simulink model "ArduCopter_3DR"  (R2015a)
settings: Solver=ode45  StartTime=0.0  StopTime=10.0  RelTol=1e-3
settings Model: CovModelRefEnable=off  Creator=pa872d  LastModifiedBy=anne

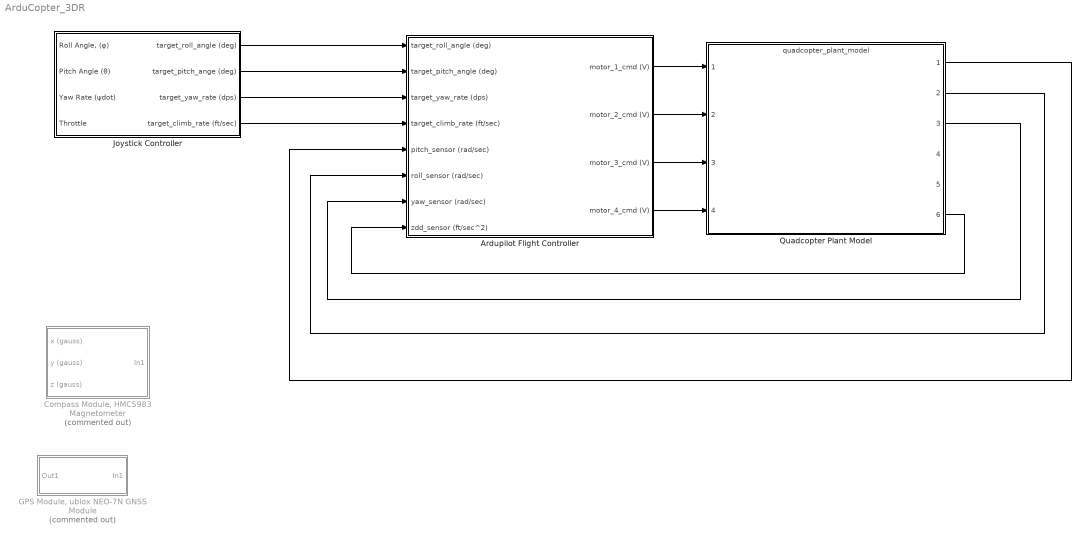
== system ArduCopter_3DR ==
  Ardupilot Flight Controller : Subsystem
  "Compass Module, HMC5983 Magnetometer" : Subsystem  Commented=on
  "GPS Module, ublox NEO-7N GNSS Module" : Subsystem  Commented=on
  Joystick Controller : Subsystem
  Quadcopter Plant Model : ModelReference  ModelNameDialog=quadcopter_plant_model.slx  SimulationMode=Normal  ModelReferenceVersion=1.2  CopyOfModelName=attitude_controller.slx  CopyOfModelName=motor_mixer.slx
  wires:
  Joystick Controller/1(target_roll_angle (deg)) -> Ardupilot Flight Controller/1(target_roll_angle (deg))
  Joystick Controller/2(target_pitch_ange (deg)) -> Ardupilot Flight Controller/2(target_pitch_angle (deg))
  Joystick Controller/3(target_yaw_rate (dps)) -> Ardupilot Flight Controller/3(target_yaw_rate (dps))
  Joystick Controller/4(target_climb_rate (ft/sec)) -> Ardupilot Flight Controller/4(target_climb_rate (ft/sec))
  Quadcopter Plant Model/1 -> Ardupilot Flight Controller/5(pitch_sensor (rad/sec))
  Quadcopter Plant Model/3 -> Ardupilot Flight Controller/7(yaw_sensor (rad/sec))
  Ardupilot Flight Controller/1(motor_1_cmd (V)) -> Quadcopter Plant Model/1
  Ardupilot Flight Controller/2(motor_2_cmd (V)) -> Quadcopter Plant Model/2
  Ardupilot Flight Controller/3(motor_3_cmd (V)) -> Quadcopter Plant Model/3
  Ardupilot Flight Controller/4(motor_4_cmd (V)) -> Quadcopter Plant Model/4
  Quadcopter Plant Model/2 -> Ardupilot Flight Controller/6(roll_sensor (rad/sec))
  Quadcopter Plant Model/6 -> Ardupilot Flight Controller/8(zdd_sensor (ft/sec^2))

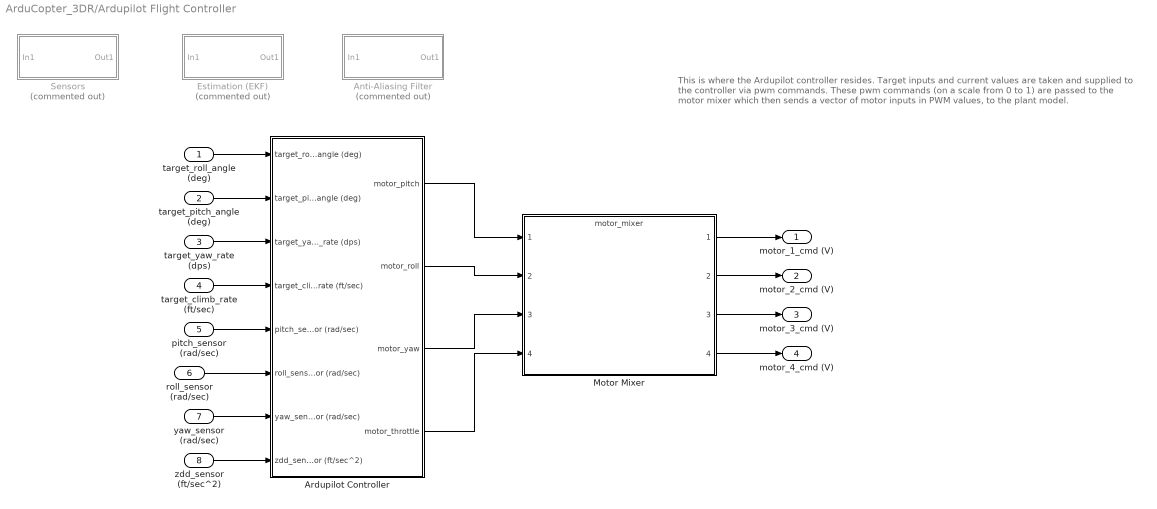
== system ArduCopter_3DR/Ardupilot Flight Controller ==
  note: This is where the Ardupilot controller resides. Target inputs and current values are taken and
      | supplied to the controller via pwm commands. These pwm commands (on a scale from 0 to 1) are passed to the motor mixer which then
      | sends a vector of motor inputs in PWM values, to the plant model.
  target_roll_angle (deg) : Inport
  target_pitch_angle (deg) : Inport  Port=2
  target_yaw_rate (dps) : Inport  Port=3
  target_climb_rate (ft/sec) : Inport  Port=4
  pitch_sensor (rad/sec) : Inport  Port=5
  roll_sensor (rad/sec) : Inport  Port=6
  yaw_sensor (rad/sec) : Inport  Port=7
  zdd_sensor (ft/sec^2) : Inport  Port=8
  Anti-Aliasing Filter : Subsystem  Commented=on
  Ardupilot Controller : Subsystem
  Estimation (EKF) : Subsystem  Commented=on
  Motor Mixer : ModelReference  ModelNameDialog=motor_mixer.slx  SimulationMode=Normal  ModelReferenceVersion=1.6  CopyOfModelName=attitude_controller.slx  CopyOfModelName=motor_mixer.slx
  Sensors : Subsystem  Commented=on
  motor_1_cmd (V) : Outport
  motor_2_cmd (V) : Outport  Port=2
  motor_3_cmd (V) : Outport  Port=3
  motor_4_cmd (V) : Outport  Port=4
  wires:
  Motor Mixer/2 -> motor_2_cmd (V)/1
  Motor Mixer/4 -> motor_4_cmd (V)/1
  Motor Mixer/3 -> motor_3_cmd (V)/1
  target_roll_angle (deg)/1 -> Ardupilot Controller/1(target_roll_angle (deg))
  target_pitch_angle (deg)/1 -> Ardupilot Controller/2(target_pitch_angle (deg))
  target_yaw_rate (dps)/1 -> Ardupilot Controller/3(target_yaw_rate (dps))
  target_climb_rate (ft/sec)/1 -> Ardupilot Controller/4(target_climb_rate (ft/sec))
  Motor Mixer/1 -> motor_1_cmd (V)/1
  yaw_sensor (rad/sec)/1 -> Ardupilot Controller/7(yaw_sensor (rad/sec))
  zdd_sensor (ft/sec^2)/1 -> Ardupilot Controller/8(zdd_sensor (ft/sec^2))
  Ardupilot Controller/1(motor_pitch) -> Motor Mixer/1
  Ardupilot Controller/2(motor_roll) -> Motor Mixer/2
  Ardupilot Controller/3(motor_yaw) -> Motor Mixer/3
  Ardupilot Controller/4(motor_throttle) -> Motor Mixer/4
  roll_sensor (rad/sec)/1 -> Ardupilot Controller/6(roll_sensor (rad/sec))
  pitch_sensor (rad/sec)/1 -> Ardupilot Controller/5(pitch_sensor (rad/sec))

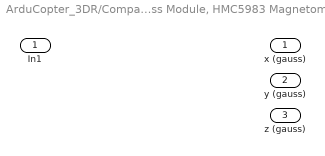
== system ArduCopter_3DR/Compass Module, HMC5983 Magnetometer ==
  In1 : Inport
  x (gauss) : Outport
  y (gauss) : Outport  Port=2
  z (gauss) : Outport  Port=3

== system ArduCopter_3DR/GPS Module, ublox NEO-7N GNSS Module ==
  In1 : Inport
  Out1 : Outport
  wires:
  In1/1 -> Out1/1

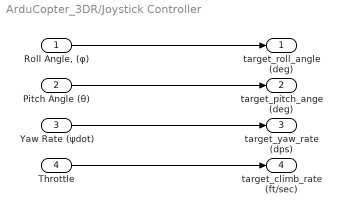
== system ArduCopter_3DR/Joystick Controller ==
  "Roll Angle, (φ)" : Inport
  Pitch Angle (θ) : Inport  Port=2
  Yaw Rate (ψdot) : Inport  Port=3
  Throttle : Inport  Port=4
  target_roll_angle (deg) : Outport
  target_pitch_ange (deg) : Outport  Port=2
  target_yaw_rate (dps) : Outport  Port=3
  target_climb_rate (ft/sec) : Outport  Port=4
  wires:
  Yaw Rate (ψdot)/1 -> target_yaw_rate (dps)/1
  Throttle/1 -> target_climb_rate (ft/sec)/1
  Pitch Angle (θ)/1 -> target_pitch_ange (deg)/1
  "Roll Angle, (φ)"/1 -> target_roll_angle (deg)/1

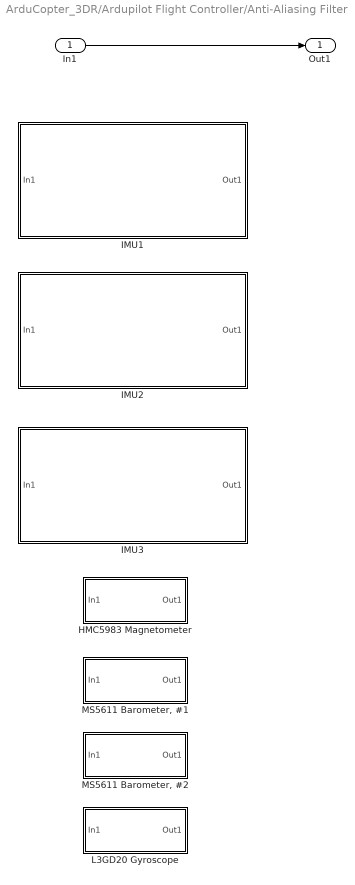
== system ArduCopter_3DR/Ardupilot Flight Controller/Anti-Aliasing Filter ==
  In1 : Inport
  HMC5983 Magnetometer : Subsystem
  IMU1 : Subsystem
  IMU2 : Subsystem
  IMU3 : Subsystem
  L3GD20 Gyroscope : Subsystem
  "MS5611 Barometer, #1" : Subsystem
  "MS5611 Barometer, #2" : Subsystem
  Out1 : Outport
  wires:
  In1/1 -> Out1/1

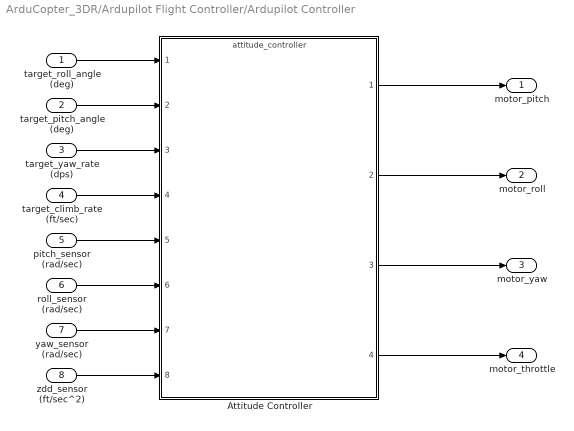
== system ArduCopter_3DR/Ardupilot Flight Controller/Ardupilot Controller ==
  target_roll_angle (deg) : Inport
  target_pitch_angle (deg) : Inport  Port=2
  target_yaw_rate (dps) : Inport  Port=3
  target_climb_rate (ft/sec) : Inport  Port=4
  pitch_sensor (rad/sec) : Inport  Port=5
  roll_sensor (rad/sec) : Inport  Port=6
  yaw_sensor (rad/sec) : Inport  Port=7
  zdd_sensor (ft/sec^2) : Inport  Port=8
  Attitude Controller : ModelReference  ModelNameDialog=attitude_controller.slx  SimulationMode=Normal  ModelReferenceVersion=1.62  CopyOfModelName=attitude_controller.slx  CopyOfModelName=motor_mixer.slx
  motor_pitch : Outport
  motor_roll : Outport  Port=2
  motor_yaw : Outport  Port=3
  motor_throttle : Outport  Port=4
  wires:
  Attitude Controller/4 -> motor_throttle/1
  Attitude Controller/3 -> motor_yaw/1
  target_roll_angle (deg)/1 -> Attitude Controller/1
  target_pitch_angle (deg)/1 -> Attitude Controller/2
  target_yaw_rate (dps)/1 -> Attitude Controller/3
  target_climb_rate (ft/sec)/1 -> Attitude Controller/4
  yaw_sensor (rad/sec)/1 -> Attitude Controller/7
  zdd_sensor (ft/sec^2)/1 -> Attitude Controller/8
  roll_sensor (rad/sec)/1 -> Attitude Controller/6
  pitch_sensor (rad/sec)/1 -> Attitude Controller/5
  Attitude Controller/2 -> motor_roll/1
  Attitude Controller/1 -> motor_pitch/1

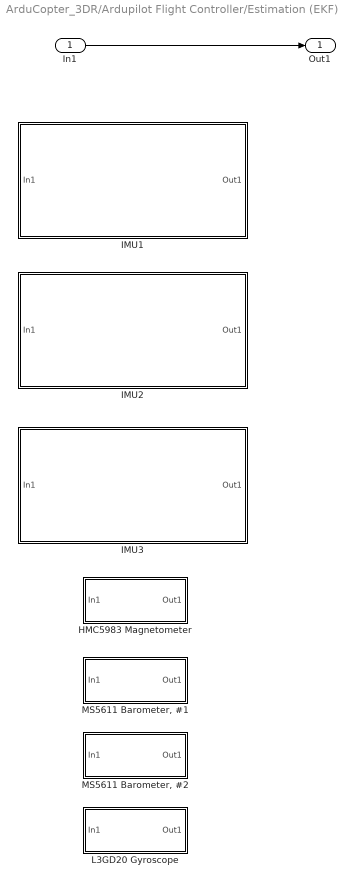
== system ArduCopter_3DR/Ardupilot Flight Controller/Estimation (EKF) ==
  In1 : Inport
  HMC5983 Magnetometer : Subsystem
  IMU1 : Subsystem
  IMU2 : Subsystem
  IMU3 : Subsystem
  L3GD20 Gyroscope : Subsystem
  "MS5611 Barometer, #1" : Subsystem
  "MS5611 Barometer, #2" : Subsystem
  Out1 : Outport
  wires:
  In1/1 -> Out1/1

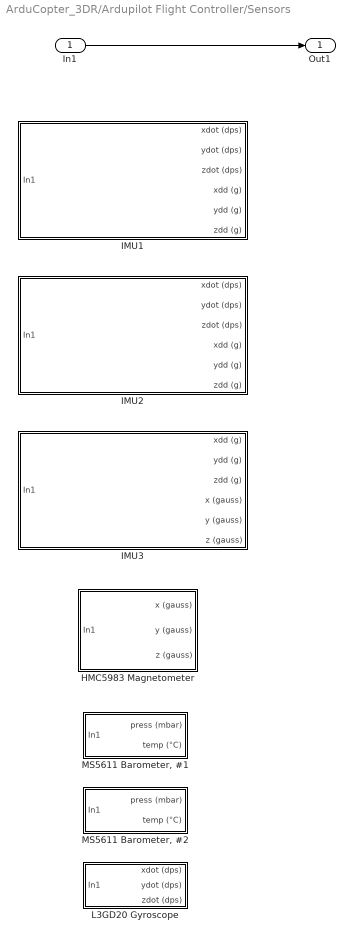
== system ArduCopter_3DR/Ardupilot Flight Controller/Sensors ==
  In1 : Inport
  HMC5983 Magnetometer : Subsystem
  IMU1 : Subsystem
  IMU2 : Subsystem
  IMU3 : Subsystem
  L3GD20 Gyroscope : Subsystem
  "MS5611 Barometer, #1" : Subsystem
  "MS5611 Barometer, #2" : Subsystem
  Out1 : Outport
  wires:
  In1/1 -> Out1/1

== system ArduCopter_3DR/Ardupilot Flight Controller/Anti-Aliasing Filter/HMC5983 Magnetometer ==
  In1 : Inport
  Out1 : Outport
  wires:
  In1/1 -> Out1/1

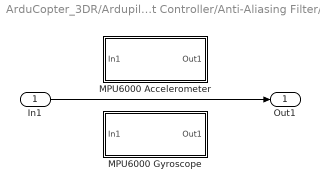
== system ArduCopter_3DR/Ardupilot Flight Controller/Anti-Aliasing Filter/IMU1 ==
  In1 : Inport
  MPU6000 Accelerometer : Subsystem
  MPU6000 Gyroscope : Subsystem
  Out1 : Outport
  wires:
  In1/1 -> Out1/1

== system ArduCopter_3DR/Ardupilot Flight Controller/Anti-Aliasing Filter/IMU2 ==
  In1 : Inport
  MPU6000 Accelerometer : Subsystem
  MPU6000 Gyroscope : Subsystem
  Out1 : Outport
  wires:
  In1/1 -> Out1/1

== system ArduCopter_3DR/Ardupilot Flight Controller/Anti-Aliasing Filter/IMU3 ==
  In1 : Inport
  LSM303D Accelerometer : Subsystem
  LSM303D Magnetometer : Subsystem
  Out1 : Outport
  wires:
  In1/1 -> Out1/1

== system ArduCopter_3DR/Ardupilot Flight Controller/Anti-Aliasing Filter/L3GD20 Gyroscope ==
  In1 : Inport
  Out1 : Outport
  wires:
  In1/1 -> Out1/1

== system ArduCopter_3DR/Ardupilot Flight Controller/Anti-Aliasing Filter/MS5611 Barometer, #1 ==
  In1 : Inport
  Out1 : Outport
  wires:
  In1/1 -> Out1/1

== system ArduCopter_3DR/Ardupilot Flight Controller/Anti-Aliasing Filter/MS5611 Barometer, #2 ==
  In1 : Inport
  Out1 : Outport
  wires:
  In1/1 -> Out1/1

== system ArduCopter_3DR/Ardupilot Flight Controller/Estimation (EKF)/HMC5983 Magnetometer ==
  In1 : Inport
  Out1 : Outport
  wires:
  In1/1 -> Out1/1

== system ArduCopter_3DR/Ardupilot Flight Controller/Estimation (EKF)/IMU1 ==
  In1 : Inport
  MPU6000 Accelerometer : Subsystem
  MPU6000 Gyroscope : Subsystem
  Out1 : Outport
  wires:
  In1/1 -> Out1/1

== system ArduCopter_3DR/Ardupilot Flight Controller/Estimation (EKF)/IMU2 ==
  In1 : Inport
  MPU6000 Accelerometer : Subsystem
  MPU6000 Gyroscope : Subsystem
  Out1 : Outport
  wires:
  In1/1 -> Out1/1

== system ArduCopter_3DR/Ardupilot Flight Controller/Estimation (EKF)/IMU3 ==
  In1 : Inport
  LSM303D Accelerometer : Subsystem
  LSM303D Magnetometer : Subsystem
  Out1 : Outport
  wires:
  In1/1 -> Out1/1

== system ArduCopter_3DR/Ardupilot Flight Controller/Estimation (EKF)/L3GD20 Gyroscope ==
  In1 : Inport
  Out1 : Outport
  wires:
  In1/1 -> Out1/1

== system ArduCopter_3DR/Ardupilot Flight Controller/Estimation (EKF)/MS5611 Barometer, #1 ==
  In1 : Inport
  Out1 : Outport
  wires:
  In1/1 -> Out1/1

== system ArduCopter_3DR/Ardupilot Flight Controller/Estimation (EKF)/MS5611 Barometer, #2 ==
  In1 : Inport
  Out1 : Outport
  wires:
  In1/1 -> Out1/1

== system ArduCopter_3DR/Ardupilot Flight Controller/Sensors/HMC5983 Magnetometer ==
  In1 : Inport
  x (gauss) : Outport
  y (gauss) : Outport  Port=2
  z (gauss) : Outport  Port=3

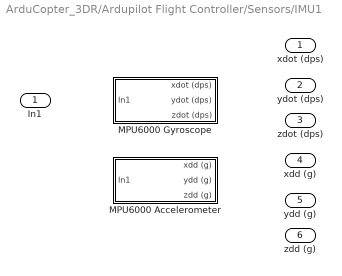
== system ArduCopter_3DR/Ardupilot Flight Controller/Sensors/IMU1 ==
  In1 : Inport
  MPU6000 Accelerometer : Subsystem
  MPU6000 Gyroscope : Subsystem
  xdot (dps) : Outport
  ydot (dps) : Outport  Port=2
  zdot (dps) : Outport  Port=3
  xdd (g) : Outport  Port=4
  ydd (g) : Outport  Port=5
  zdd (g) : Outport  Port=6

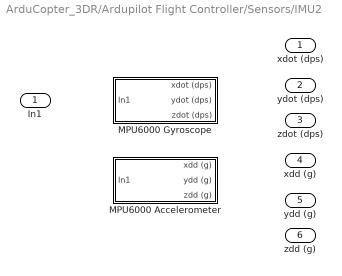
== system ArduCopter_3DR/Ardupilot Flight Controller/Sensors/IMU2 ==
  In1 : Inport
  MPU6000 Accelerometer : Subsystem
  MPU6000 Gyroscope : Subsystem
  xdot (dps) : Outport
  ydot (dps) : Outport  Port=2
  zdot (dps) : Outport  Port=3
  xdd (g) : Outport  Port=4
  ydd (g) : Outport  Port=5
  zdd (g) : Outport  Port=6

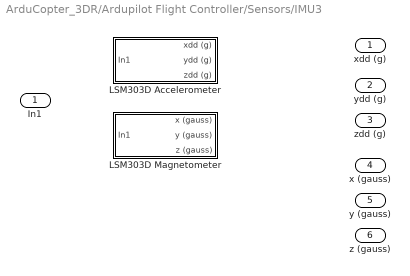
== system ArduCopter_3DR/Ardupilot Flight Controller/Sensors/IMU3 ==
  In1 : Inport
  LSM303D Accelerometer : Subsystem
  LSM303D Magnetometer : Subsystem
  xdd (g) : Outport
  ydd (g) : Outport  Port=2
  zdd (g) : Outport  Port=3
  x (gauss) : Outport  Port=4
  y (gauss) : Outport  Port=5
  z (gauss) : Outport  Port=6

== system ArduCopter_3DR/Ardupilot Flight Controller/Sensors/L3GD20 Gyroscope ==
  In1 : Inport
  xdot (dps) : Outport
  ydot (dps) : Outport  Port=2
  zdot (dps) : Outport  Port=3

== system ArduCopter_3DR/Ardupilot Flight Controller/Sensors/MS5611 Barometer, #1 ==
  In1 : Inport
  press (mbar) : Outport
  temp (°C) : Outport  Port=2

== system ArduCopter_3DR/Ardupilot Flight Controller/Sensors/MS5611 Barometer, #2 ==
  In1 : Inport
  press (mbar) : Outport
  temp (°C) : Outport  Port=2

== system ArduCopter_3DR/Ardupilot Flight Controller/Anti-Aliasing Filter/IMU1/MPU6000 Accelerometer ==
  In1 : Inport
  Out1 : Outport
  wires:
  In1/1 -> Out1/1

== system ArduCopter_3DR/Ardupilot Flight Controller/Anti-Aliasing Filter/IMU1/MPU6000 Gyroscope ==
  In1 : Inport
  Out1 : Outport
  wires:
  In1/1 -> Out1/1

== system ArduCopter_3DR/Ardupilot Flight Controller/Anti-Aliasing Filter/IMU2/MPU6000 Accelerometer ==
  In1 : Inport
  Out1 : Outport
  wires:
  In1/1 -> Out1/1

== system ArduCopter_3DR/Ardupilot Flight Controller/Anti-Aliasing Filter/IMU2/MPU6000 Gyroscope ==
  In1 : Inport
  Out1 : Outport
  wires:
  In1/1 -> Out1/1

== system ArduCopter_3DR/Ardupilot Flight Controller/Anti-Aliasing Filter/IMU3/LSM303D Accelerometer ==
  In1 : Inport
  Out1 : Outport
  wires:
  In1/1 -> Out1/1

== system ArduCopter_3DR/Ardupilot Flight Controller/Anti-Aliasing Filter/IMU3/LSM303D Magnetometer ==
  In1 : Inport
  Out1 : Outport
  wires:
  In1/1 -> Out1/1

== system ArduCopter_3DR/Ardupilot Flight Controller/Estimation (EKF)/IMU1/MPU6000 Accelerometer ==
  In1 : Inport
  Out1 : Outport
  wires:
  In1/1 -> Out1/1

== system ArduCopter_3DR/Ardupilot Flight Controller/Estimation (EKF)/IMU1/MPU6000 Gyroscope ==
  In1 : Inport
  Out1 : Outport
  wires:
  In1/1 -> Out1/1

== system ArduCopter_3DR/Ardupilot Flight Controller/Estimation (EKF)/IMU2/MPU6000 Accelerometer ==
  In1 : Inport
  Out1 : Outport
  wires:
  In1/1 -> Out1/1

== system ArduCopter_3DR/Ardupilot Flight Controller/Estimation (EKF)/IMU2/MPU6000 Gyroscope ==
  In1 : Inport
  Out1 : Outport
  wires:
  In1/1 -> Out1/1

== system ArduCopter_3DR/Ardupilot Flight Controller/Estimation (EKF)/IMU3/LSM303D Accelerometer ==
  In1 : Inport
  Out1 : Outport
  wires:
  In1/1 -> Out1/1

== system ArduCopter_3DR/Ardupilot Flight Controller/Estimation (EKF)/IMU3/LSM303D Magnetometer ==
  In1 : Inport
  Out1 : Outport
  wires:
  In1/1 -> Out1/1

== system ArduCopter_3DR/Ardupilot Flight Controller/Sensors/IMU1/MPU6000 Accelerometer ==
  In1 : Inport
  xdd (g) : Outport
  ydd (g) : Outport  Port=2
  zdd (g) : Outport  Port=3

== system ArduCopter_3DR/Ardupilot Flight Controller/Sensors/IMU1/MPU6000 Gyroscope ==
  In1 : Inport
  xdot (dps) : Outport
  ydot (dps) : Outport  Port=2
  zdot (dps) : Outport  Port=3

== system ArduCopter_3DR/Ardupilot Flight Controller/Sensors/IMU2/MPU6000 Accelerometer ==
  In1 : Inport
  xdd (g) : Outport
  ydd (g) : Outport  Port=2
  zdd (g) : Outport  Port=3

== system ArduCopter_3DR/Ardupilot Flight Controller/Sensors/IMU2/MPU6000 Gyroscope ==
  In1 : Inport
  xdot (dps) : Outport
  ydot (dps) : Outport  Port=2
  zdot (dps) : Outport  Port=3

== system ArduCopter_3DR/Ardupilot Flight Controller/Sensors/IMU3/LSM303D Accelerometer ==
  In1 : Inport
  xdd (g) : Outport
  ydd (g) : Outport  Port=2
  zdd (g) : Outport  Port=3

== system ArduCopter_3DR/Ardupilot Flight Controller/Sensors/IMU3/LSM303D Magnetometer ==
  In1 : Inport
  x (gauss) : Outport
  y (gauss) : Outport  Port=2
  z (gauss) : Outport  Port=3
